simulink library "ThrusterAllocation"  (R2013a)
settings: Solver=ode3  StartTime=0.0  StopTime=10.0  RelTol=1e-3
undefined symbols (not defined in the file): nSwitchboard, nThrusters, singularityAvoidanceCostGain, singularityAvoidanceCostSmoother, TA_sampling_time, thrustAllocationSamplingTime
settings Model: Creator=torstebo  LastModifiedBy=torstebo

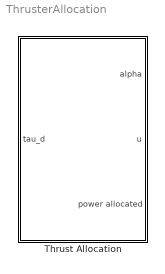
== system ThrusterAllocation ==
  Thrust Allocation : Subsystem  SystemSampleTime=TA_sampling_time

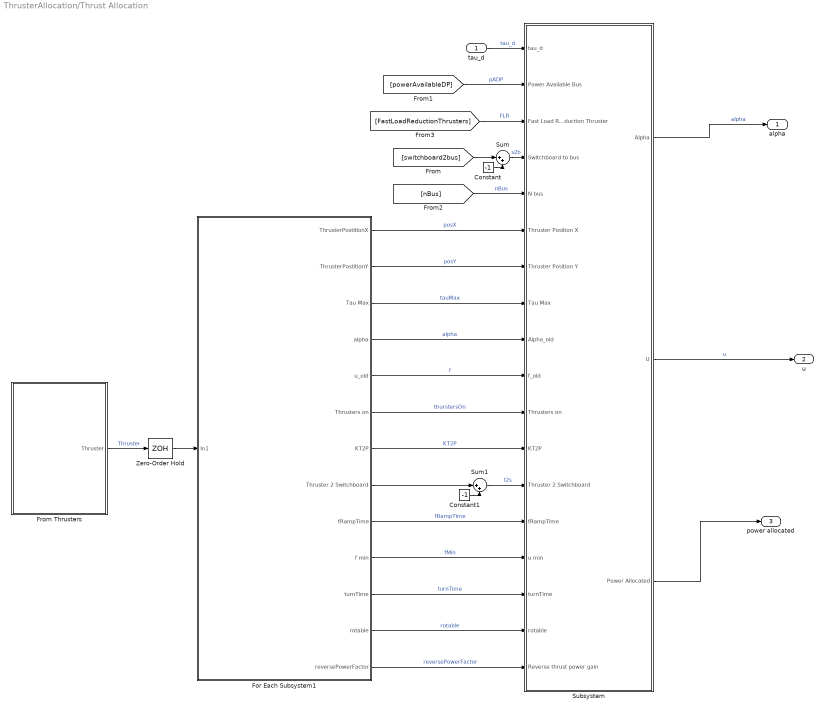
== system ThrusterAllocation/Thrust Allocation ==
  tau_d : Inport
  Constant : Constant  Value=-1
  Constant1 : Constant  Value=-1
  For Each Subsystem1 : Subsystem  TreatAsAtomicUnit=on
  From Thrusters : Subsystem  Tag=ThrusterAllocation/FromThrusters
  Subsystem : Subsystem
  Sum : Sum  Inputs=|++
  Sum1 : Sum  Inputs=|++
  Zero-Order Hold : ZeroOrderHold  SampleTime=thrustAllocationSamplingTime
  alpha : Outport
  u : Outport  Port=2
  power allocated : Outport  Port=3
  wires:
  For Each Subsystem1/11(turnTime) -> Subsystem/16(turnTime)  "turnTime"
  For Each Subsystem1/7(KT2P) -> Subsystem/12(KT2P)  "KT2P"
  For Each Subsystem1/6(Thrusters on) -> Subsystem/11(Thrusters on)  "thurstersOn"
  For Each Subsystem1/5(u_old) -> Subsystem/10(f_old)  "f"
  For Each Subsystem1/4(alpha) -> Subsystem/9(Alpha_old)  "alpha"
  For Each Subsystem1/3(Tau Max) -> Subsystem/8(Tau Max)  "tauMax"
  For Each Subsystem1/2(ThrusterPostitionY) -> Subsystem/7(Thruster Position Y)  "posY"
  For Each Subsystem1/1(ThrusterPostitionX) -> Subsystem/6(Thruster Position X)  "posX"
  [nBus] -> Subsystem/5(N bus)  "nBus"
  Sum/1 -> Subsystem/4(Switchboard to bus)  "s2b"
  tau_d/1 -> Subsystem/1(tau_d)  "tau_d"
  Constant/1 -> Sum/2
  [switchboard2bus] -> Sum/1
  From Thrusters/1(Thruster) -> Zero-Order Hold/1  "Thruster"
  Sum1/1 -> Subsystem/13(Thruster 2 Switchboard)  "t2s"
  Constant1/1 -> Sum1/2
  For Each Subsystem1/8(Thruster 2 Switchboard) -> Sum1/1
  For Each Subsystem1/9(fRampTime) -> Subsystem/14(fRampTime)  "fRampTime"
  For Each Subsystem1/10(f min) -> Subsystem/15(u min)  "fMin"
  For Each Subsystem1/12(rotable) -> Subsystem/17(rotable)  "rotable"
  For Each Subsystem1/13(reversePowerFactor) -> Subsystem/18(Reverse thrust power gain)  "reversePowerFactor"
  [FastLoadReductionThrusters] -> Subsystem/3(Fast Load Reduction Thruster)  "FLR"
  Zero-Order Hold/1 -> For Each Subsystem1/1(In1)
  [powerAvailableDP] -> Subsystem/2(Power Available Bus)  "pADP"
  Subsystem/2(U) -> u/1  "u"
  Subsystem/3(Power Allocated) -> power allocated/1
  Subsystem/1(Alpha) -> alpha/1  "alpha"

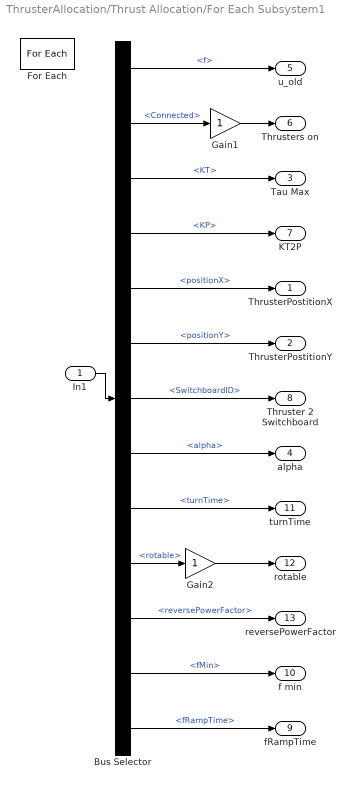
== system ThrusterAllocation/Thrust Allocation/For Each Subsystem1 ==
  In1 : Inport  OutDataTypeStr=Bus: ThrusterBus  Partition=on  PartitionDimension=1  PartitionWidth=1
  Bus Selector : BusSelector  OutputSignals=f,Connected,KT,KP,positionX,positionY,SwitchboardID,alpha,turnTime,rotable,reversePowerFactor,fMin,fRampTime
  For Each : ForEach  DisableCoverage=on  IndexMode=One-based
  Gain1 : Gain  OutDataTypeStr=double
  Gain2 : Gain  OutDataTypeStr=double
  ThrusterPostitionX : Outport  ConcatenationDimension=1
  ThrusterPostitionY : Outport  Port=2  ConcatenationDimension=1
  Tau Max : Outport  Port=3  ConcatenationDimension=1
  alpha : Outport  Port=4  ConcatenationDimension=1
  u_old : Outport  Port=5  ConcatenationDimension=1
  Thrusters on : Outport  Port=6  ConcatenationDimension=1
  KT2P : Outport  Port=7  ConcatenationDimension=1
  Thruster 2 Switchboard : Outport  Port=8  ConcatenationDimension=1
  fRampTime : Outport  Port=9  ConcatenationDimension=1
  f min : Outport  Port=10  ConcatenationDimension=1
  turnTime : Outport  Port=11  ConcatenationDimension=1
  rotable : Outport  Port=12  ConcatenationDimension=1
  reversePowerFactor : Outport  Port=13  ConcatenationDimension=1
  wires:
  Bus Selector/13 -> fRampTime/1  "<fRampTime>"
  Bus Selector/12 -> f min/1  "<fMin>"
  Bus Selector/11 -> reversePowerFactor/1  "<reversePowerFactor>"
  Bus Selector/9 -> turnTime/1  "<turnTime>"
  Bus Selector/10 -> Gain2/1  "<rotable>"
  Bus Selector/8 -> alpha/1  "<alpha>"
  Bus Selector/7 -> Thruster 2 Switchboard/1  "<SwitchboardID>"
  Bus Selector/6 -> ThrusterPostitionY/1  "<positionY>"
  Bus Selector/5 -> ThrusterPostitionX/1  "<positionX>"
  Gain1/1 -> Thrusters on/1
  Bus Selector/4 -> KT2P/1  "<KP>"
  Bus Selector/3 -> Tau Max/1  "<KT>"
  Bus Selector/2 -> Gain1/1  "<Connected>"
  Bus Selector/1 -> u_old/1  "<f>"
  In1/1 -> Bus Selector/1
  Gain2/1 -> rotable/1

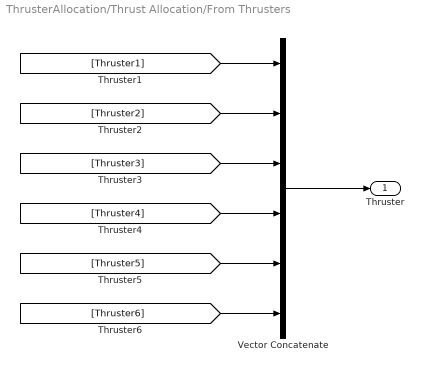
== system ThrusterAllocation/Thrust Allocation/From Thrusters ==
  Vector Concatenate : Concatenate  Tag=FromThrusters/Merger  NumInputs=6
  Thruster : Outport
  wires:
  Vector Concatenate/1 -> Thruster/1
  [Thruster1] -> Vector Concatenate/1
  [Thruster2] -> Vector Concatenate/2
  [Thruster3] -> Vector Concatenate/3
  [Thruster4] -> Vector Concatenate/4
  [Thruster5] -> Vector Concatenate/5
  [Thruster6] -> Vector Concatenate/6

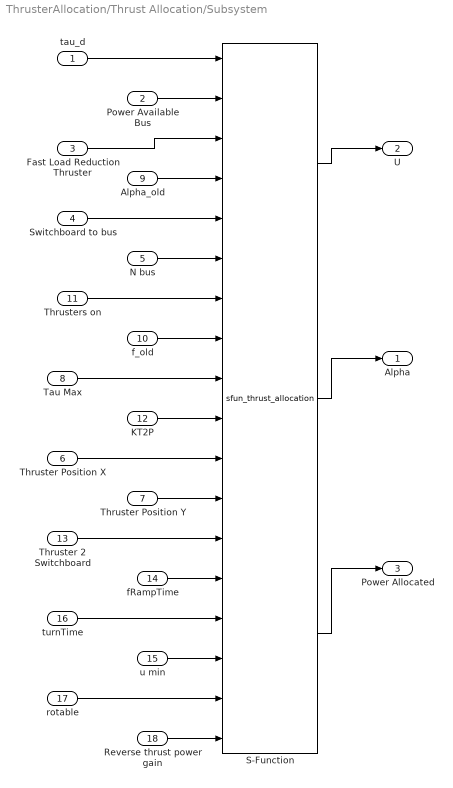
== system ThrusterAllocation/Thrust Allocation/Subsystem ==
  tau_d : Inport
  Power Available Bus : Inport  Port=2
  Fast Load Reduction Thruster : Inport  Port=3
  Switchboard to bus : Inport  Port=4
  N bus : Inport  Port=5
  Thruster Position X : Inport  Port=6
  Thruster Position Y : Inport  Port=7
  Tau Max : Inport  Port=8
  Alpha_old : Inport  Port=9
  f_old : Inport  Port=10
  Thrusters on : Inport  Port=11
  KT2P : Inport  Port=12
  Thruster 2 Switchboard : Inport  Port=13
  fRampTime : Inport  Port=14
  u min : Inport  Port=15
  turnTime : Inport  Port=16
  rotable : Inport  Port=17
  Reverse thrust power gain : Inport  Port=18
  S-Function : S-Function  FunctionName=sfun_thrust_allocation  Parameters=thrustAllocationSamplingTime,nThrusters,nSwitchboard,singularityAvoidanceCostGain,singularityAvoidanceCostSmoother  EnableBusSupport=off
  Alpha : Outport
  U : Outport  Port=2
  Power Allocated : Outport  Port=3
  wires:
  f_old/1 -> S-Function/8
  Thrusters on/1 -> S-Function/7
  N bus/1 -> S-Function/6
  Switchboard to bus/1 -> S-Function/5
  Alpha_old/1 -> S-Function/4
  Fast Load Reduction Thruster/1 -> S-Function/3
  tau_d/1 -> S-Function/1
  Power Available Bus/1 -> S-Function/2
  S-Function/1 -> U/1
  S-Function/2 -> Alpha/1
  turnTime/1 -> S-Function/15
  fRampTime/1 -> S-Function/14
  Thruster 2 Switchboard/1 -> S-Function/13
  Thruster Position Y/1 -> S-Function/12
  Thruster Position X/1 -> S-Function/11
  KT2P/1 -> S-Function/10
  Tau Max/1 -> S-Function/9
  u min/1 -> S-Function/16
  S-Function/3 -> Power Allocated/1
  rotable/1 -> S-Function/17
  Reverse thrust power gain/1 -> S-Function/18
